simulink model "spacecraft_model_old"  (R2017a)
settings: Solver=VariableStepAuto  StartTime=0.0  StopTime=sim_time  RelTol=1e-3
StopFcn:
  | start_animation
values from neighbouring files (symbols this model uses):
  Ap = 0.1*0.2    (= 0.02)    [main_old.m]    (also in setup.m)
  Cd = 2.0    (= 2)    [main_old.m]    (also in mon_main.m = 2.2; orbit.m = 2.2; setup.m)
  Cp = 1.6    [main_old.m]    (also in setup.m)
  g_chap = q_chap(1:3)'    [main_old.m]    (also in setup.m = [0 0 0]; start_simulation_old.m)
  g_chap_data = []    [main_old.m]    (also in start_simulation_old.m)
  h_0 = [0,0,0]'    [main_old.m]    (also in setup.m)
  h_chap = [0.01 0.01 0.01]    [main_old.m]    (also in main_old2.m = [.0005;.0005;.0005]; setup.m)
  I = diag([I_x,I_y,I_z])    [main_old.m]    (also in setup.m)
  i_max = 0.25    [main_old.m]    (also in setup.m)
  K_data = []    [main_old.m]    (also in start_simulation_old.m)
  m_dipoleDist = [0.0001; -0.0001; 0.0005]'    [main_old.m]    (also in setup.m)
  mx_max = 0.2    [main_old.m]    (also in setup.m)
  my_max = 0.2    [main_old.m]    (also in setup.m)
  mz_max = 0.2    [main_old.m]    (also in setup.m)
  Pp = 4.5*10^-6    (= 4.5e-06)    [main_old.m]    (also in setup.m)
  q_0 = euler2quat(euler_0)'    [main_old.m]    (also in setup.m; start_simulation_old.m = euler2quat(euler_o_b_0)')
  r = 1+k    [anim_old.m]    (also in main_old.m = [0.005,0.001,0.001]'; orbit_J2.m = norm(y(1:3)); orbit_spherical.m = norm(y(1:3)); setup.m = [0.005,0.001,0.001]')
  rho = 42.418*10^-11    (= 4.2418e-10)    [main_old.m]    (also in mon_main.m = 2.6e-12; orbit.m = 2.6e-12; setup.m)
  sample_time = step_time*lqr_step    (= 0.1)    [main_old.m]    (also in start_simulation_old.m = 1)
  v0 = 2*pi*r_o/T_o    [main_old.m]    (also in setup.m)
  vx_max = 2.5    [main_old.m]    (also in setup.m)
  vy_max = 2.5    [main_old.m]    (also in setup.m)
  vz_max = 5    [main_old.m]    (also in setup.m)
  W = wheels_config.distr_matrix    [main_old.m]    (also in setup.m)
  w_0 = sqrt(mu/(r_o^3))    [main_old.m]    (also in setup.m)
  w_b_ib_0 = w0 + w_o_ib    [main_old.m]    (also in setup.m; start_simulation_old.m = w_o_b_0 + w_o_ib)
  w_chap = [0 0 0]    [main_old.m]    (also in main_old2.m = [0;0;0]; setup.m)
  w_o_io = [0,w_0,0]'    [main_old.m]    (also in setup.m; start_simulation_old.m = [0;w_0;0])
undefined symbols (not defined in the file or in its folder): box300, boy300, boz300, C, Ki, Kr, time300
libraries: vrlib x6, simulink x1
settings Model: Creator=Araawn  LastModifiedBy=Araawn

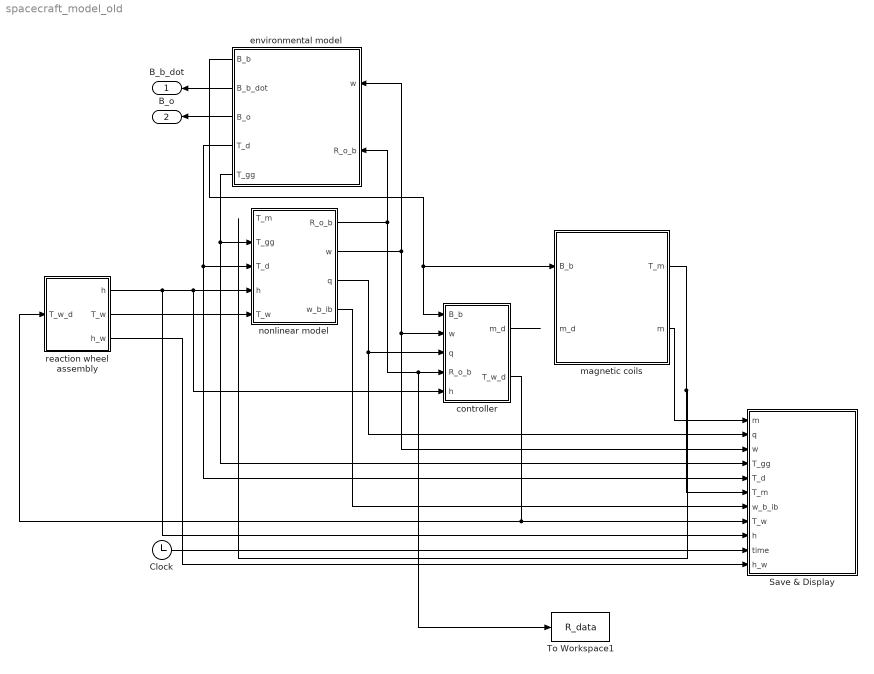
== system spacecraft_model_old ==
  Clock : Clock
  Save & Display : Subsystem
  To Workspace1 : ToWorkspace  VariableName=R_data  SaveFormat=Timeseries  SampleTime=-1
  controller : Subsystem
  environmental model : Subsystem
  magnetic coils : Subsystem
  "nonlinear model " : Subsystem
  reaction wheel assembly : Subsystem
  B_b_dot : Outport
  B_o : Outport  Port=2
  wires:
  environmental model/5(T_gg) -> "nonlinear model "/2("T_gg "), Save & Display/4(T_gg)
  environmental model/4(T_d) -> "nonlinear model "/3(T_d), Save & Display/5(T_d)
  "nonlinear model "/2(w) -> environmental model/1(w), Save & Display/3(w), controller/2(w)
  "nonlinear model "/1(R_o_b) -> To Workspace1/1, controller/4(R_o_b), environmental model/2(R_o_b)
  Clock/1 -> Save & Display/10(time)
  "nonlinear model "/3("q ") -> Save & Display/2(q), controller/3(q)
  environmental model/3(B_o) -> B_o/1
  environmental model/2(B_b_dot) -> B_b_dot/1
  "nonlinear model "/4(w_b_ib) -> Save & Display/7(w_b_ib)
  reaction wheel assembly/1(h) -> Save & Display/9(h), "nonlinear model "/4(h), controller/5(h)
  controller/2(T_w_d) -> reaction wheel assembly/1(T_w_d), Save & Display/8(T_w)
  magnetic coils/2(m) -> Save & Display/1(m)
  environmental model/1(B_b) -> magnetic coils/1(B_b), controller/1(B_b)
  controller/1(m_d) -> ?
  magnetic coils/1(T_m) -> Save & Display/6(T_m)
  reaction wheel assembly/2(T_w) -> "nonlinear model "/5(T_w)
  reaction wheel assembly/3(h_w) -> Save & Display/11(h_w)

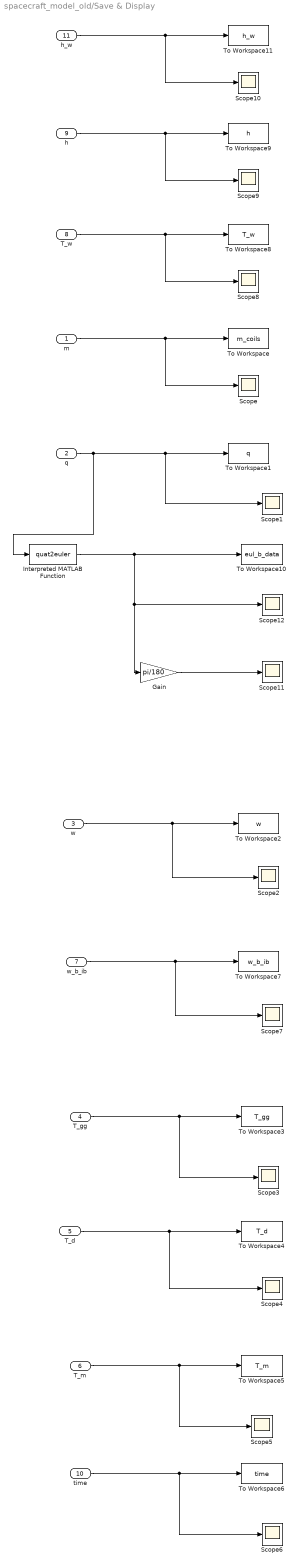
== system spacecraft_model_old/Save & Display ==
  m : Inport
  q : Inport  Port=2
  w : Inport  Port=3
  T_gg : Inport  Port=4
  T_d : Inport  Port=5
  T_m : Inport  Port=6
  w_b_ib : Inport  Port=7
  T_w : Inport  Port=8
  h : Inport  Port=9
  time : Inport  Port=10
  h_w : Inport  Port=11
  Gain : Gain  Gain=pi/180
  Interpreted MATLAB Function : MATLABFcn  MATLABFcn=quat2euler
  Scope{,1..12} (13 alike) : Scope
  To Workspace : ToWorkspace  VariableName=m_coils  SaveFormat=Timeseries  SampleTime=-1
  To Workspace1 : ToWorkspace  VariableName=q  SaveFormat=Timeseries  SampleTime=-1
  To Workspace10 : ToWorkspace  VariableName=eul_b_data  SaveFormat=Timeseries  SampleTime=-1
  To Workspace11 : ToWorkspace  VariableName=h_w  SaveFormat=Timeseries  SampleTime=-1
  To Workspace2 : ToWorkspace  VariableName=w  SaveFormat=Timeseries  SampleTime=-1
  To Workspace3 : ToWorkspace  VariableName=T_gg  SaveFormat=Timeseries  SampleTime=-1
  To Workspace4 : ToWorkspace  VariableName=T_d  SaveFormat=Timeseries  SampleTime=-1
  To Workspace5 : ToWorkspace  VariableName=T_m  SaveFormat=Timeseries  SampleTime=-1
  To Workspace6 : ToWorkspace  VariableName=time  SaveFormat=Timeseries  SampleTime=-1
  To Workspace7 : ToWorkspace  VariableName=w_b_ib  SaveFormat=Timeseries  SampleTime=-1
  To Workspace8 : ToWorkspace  VariableName=T_w  SaveFormat=Timeseries  SampleTime=-1
  To Workspace9 : ToWorkspace  VariableName=h  SaveFormat=Timeseries  SampleTime=-1
  wires:
  m/1 -> Scope/1, To Workspace/1
  q/1 -> Interpreted MATLAB Function/1, Scope1/1, To Workspace1/1
  w/1 -> Scope2/1, To Workspace2/1
  T_gg/1 -> Scope3/1, To Workspace3/1
  T_d/1 -> Scope4/1, To Workspace4/1
  T_m/1 -> Scope5/1, To Workspace5/1
  time/1 -> Scope6/1, To Workspace6/1
  w_b_ib/1 -> Scope7/1, To Workspace7/1
  T_w/1 -> Scope8/1, To Workspace8/1
  h/1 -> Scope9/1, To Workspace9/1
  Interpreted MATLAB Function/1 -> To Workspace10/1, Scope12/1, Gain/1
  Gain/1 -> Scope11/1
  h_w/1 -> Scope10/1, To Workspace11/1

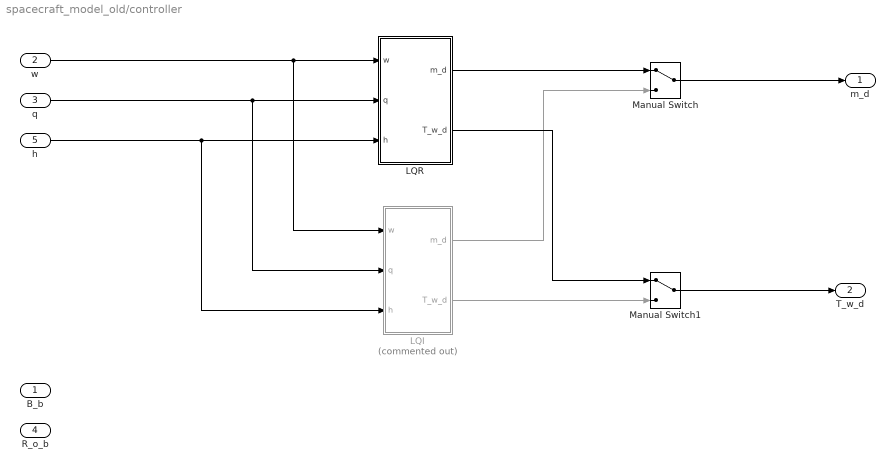
== system spacecraft_model_old/controller ==
  B_b : Inport
  w : Inport  Port=2
  q : Inport  Port=3
  R_o_b : Inport  Port=4
  h : Inport  Port=5
  LQI : Subsystem  Commented=on
  LQR : Subsystem
  Manual Switch : ManualSwitch
  Manual Switch1 : ManualSwitch
  m_d : Outport
  T_w_d : Outport  Port=2
  wires:
  w/1 -> LQR/1(w), LQI/1(w)
  q/1 -> LQR/2(q), LQI/2(q)
  h/1 -> LQR/3(h), LQI/3(h)
  LQR/1(m_d) -> Manual Switch/1
  LQI/1(m_d) -> Manual Switch/2
  Manual Switch/1 -> m_d/1
  LQI/2(T_w_d) -> Manual Switch1/2
  LQR/2(T_w_d) -> Manual Switch1/1
  Manual Switch1/1 -> T_w_d/1

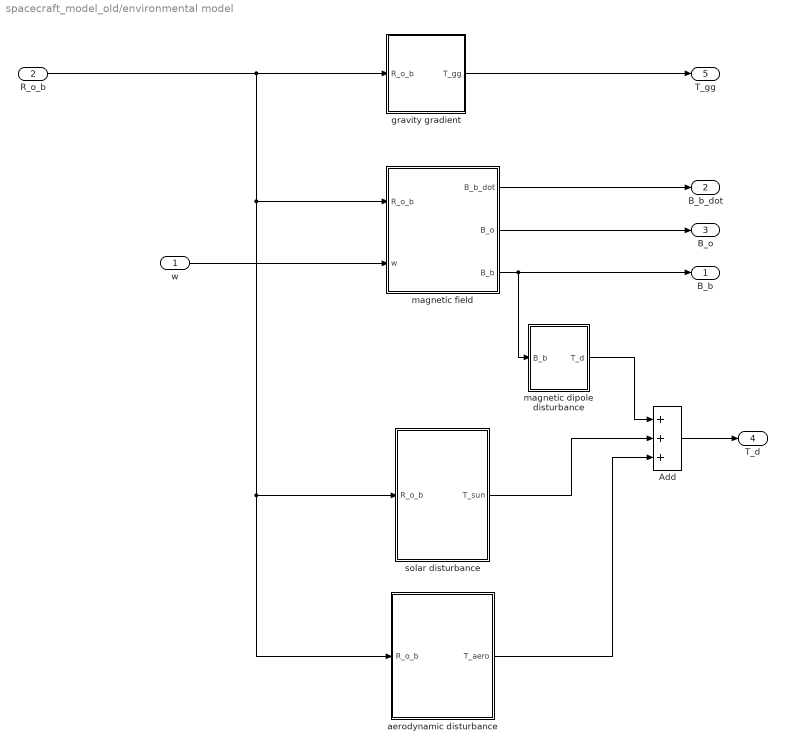
== system spacecraft_model_old/environmental model ==
  w : Inport
  R_o_b : Inport  Port=2
  Add : Sum  Inputs=+++
  aerodynamic disturbance : Subsystem
  gravity gradient : Subsystem
  magnetic dipole disturbance : Subsystem
  magnetic field : Subsystem
  solar disturbance : Subsystem
  B_b : Outport
  B_b_dot : Outport  Port=2
  B_o : Outport  Port=3
  T_d : Outport  Port=4
  T_gg : Outport  Port=5
  wires:
  magnetic field/3(B_b) -> B_b/1, magnetic dipole disturbance/1(B_b)
  Add/1 -> T_d/1
  magnetic dipole disturbance/1(T_d) -> Add/1
  magnetic field/2(B_o) -> B_o/1
  gravity gradient/1(T_gg) -> T_gg/1
  solar disturbance/1(T_sun) -> Add/2
  aerodynamic disturbance/1(T_aero) -> Add/3
  magnetic field/1(B_b_dot) -> B_b_dot/1
  R_o_b/1 -> gravity gradient/1(R_o_b), solar disturbance/1(R_o_b), aerodynamic disturbance/1(R_o_b), magnetic field/1(R_o_b)
  w/1 -> magnetic field/2(w)

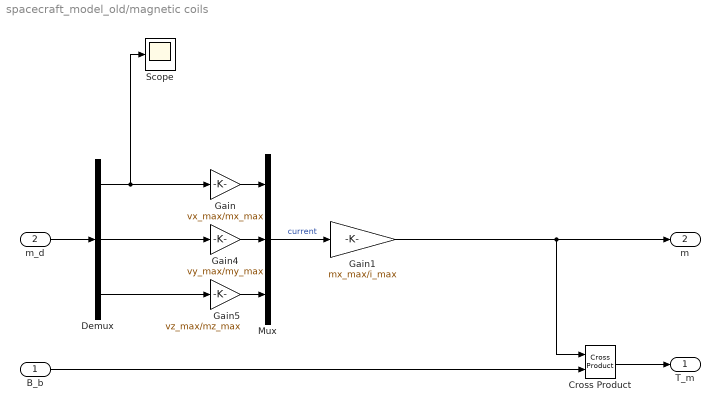
== system spacecraft_model_old/magnetic coils ==
  B_b : Inport
  m_d : Inport  Port=2
  Cross Product : vrlib/Utilities/Cross Product
      settings: SourceProductBaseCode=VR
  Demux : Demux  Outputs=3
  Gain : Gain  Gain=vx_max/mx_max
  Gain1 : Gain  Gain=mx_max/i_max
  Gain4 : Gain  Gain=vy_max/my_max
  Gain5 : Gain  Gain=vz_max/mz_max
  Mux : Mux  Inputs=3
  Scope : Scope
  T_m : Outport
  m : Outport  Port=2
  wires:
  Demux/1 -> Gain/1, Scope/1
  B_b/1 -> Cross Product/2
  Mux/1 -> Gain1/1  "current"
  Demux/3 -> Gain5/1
  Cross Product/1 -> T_m/1
  Demux/2 -> Gain4/1
  m_d/1 -> Demux/1
  Gain1/1 -> m/1, Cross Product/1
  Gain/1 -> Mux/1
  Gain5/1 -> Mux/3
  Gain4/1 -> Mux/2

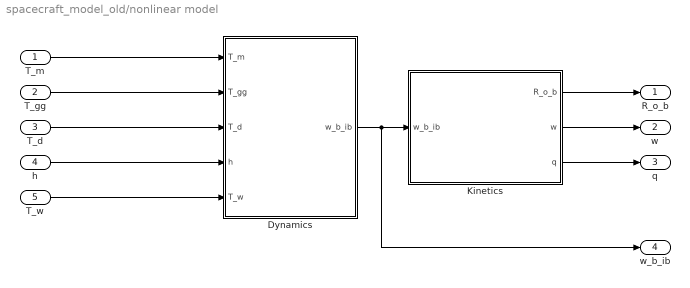
== system spacecraft_model_old/nonlinear model  ==
  T_m : Inport
  "T_gg " : Inport  Port=2
  T_d : Inport  Port=3
  h : Inport  Port=4
  T_w : Inport  Port=5
  "Dynamics " : Subsystem
  Kinetics : Subsystem
  R_o_b : Outport
  w : Outport  Port=2
  "q " : Outport  Port=3
  w_b_ib : Outport  Port=4
  wires:
  T_m/1 -> "Dynamics "/1(T_m)
  "T_gg "/1 -> "Dynamics "/2(T_gg)
  T_d/1 -> "Dynamics "/3(T_d)
  Kinetics/3(q) -> "q "/1
  Kinetics/1(R_o_b) -> R_o_b/1
  Kinetics/2(w) -> w/1
  "Dynamics "/1(w_b_ib) -> Kinetics/1("w_b_ib "), w_b_ib/1
  h/1 -> "Dynamics "/4(h)
  T_w/1 -> "Dynamics "/5(T_w)

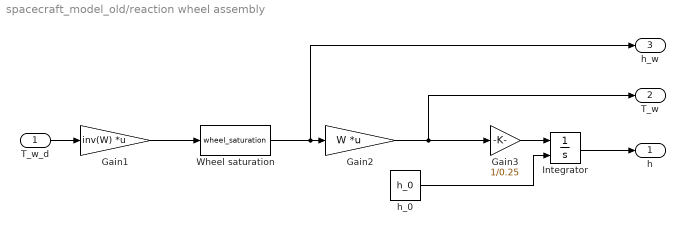
== system spacecraft_model_old/reaction wheel assembly ==
  T_w_d : Inport
  Gain1 : Gain  Gain=inv(W)  Multiplication=Matrix(K*u)
  Gain2 : Gain  Gain=W  Multiplication=Matrix(K*u)
  Gain3 : Gain  Gain=1/0.25
  Integrator : Integrator  InitialConditionSource=external
  Wheel saturation : MATLABFcn  MATLABFcn=wheel_saturation  Output1D=off
  h_0 : Constant  Value=h_0  VectorParams1D=off
  h : Outport
  T_w : Outport  Port=2
  h_w : Outport  Port=3
  wires:
  T_w_d/1 -> Gain1/1
  Gain3/1 -> Integrator/1
  h_0/1 -> Integrator/2
  Integrator/1 -> h/1
  Wheel saturation/1 -> h_w/1, Gain2/1
  Gain2/1 -> Gain3/1, T_w/1
  Gain1/1 -> Wheel saturation/1

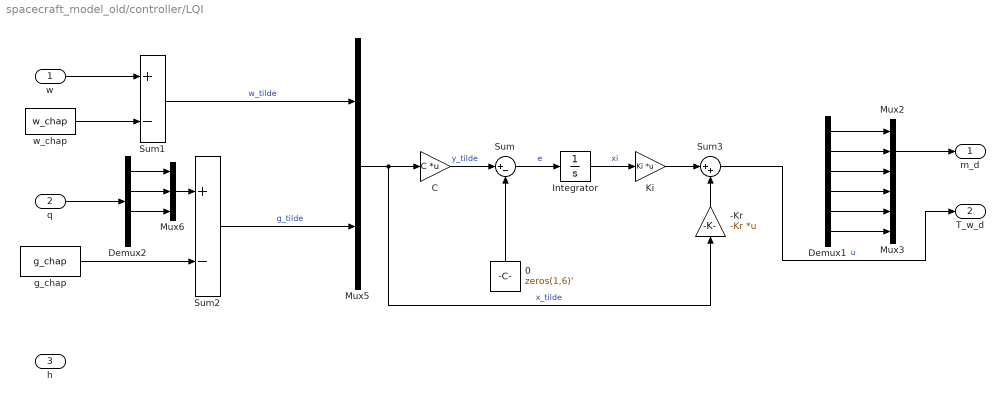
== system spacecraft_model_old/controller/LQI ==
  w : Inport
  q : Inport  Port=2
  h : Inport  Port=3
  -Kr : Gain  Gain=-Kr  Multiplication=Matrix(K*u)
  0 : Constant  Value=zeros(1,6)'
  C : Gain  Gain=C  Multiplication=Matrix(K*u)
  Demux1 : Demux  Outputs=6
  Demux2 : Demux
  Integrator : Integrator
  Ki : Gain  Gain=Ki  Multiplication=Matrix(K*u)
  Mux2 : Mux  Inputs=3
  Mux3 : Mux  Inputs=3
  Mux5 : Mux  Inputs=2
  Mux6 : Mux  Inputs=3
  Sum : Sum  Inputs=|+-
  Sum1 : Sum  Inputs=+-
  Sum2 : Sum  Inputs=+-
  Sum3 : Sum  Inputs=|++
  g_chap : Constant  Value=g_chap
  w_chap : Constant  Value=w_chap
  m_d : Outport
  T_w_d : Outport  Port=2
  wires:
  w/1 -> Sum1/1
  q/1 -> Demux2/1
  Demux1/1 -> Mux2/1
  Demux1/2 -> Mux2/2
  Demux1/3 -> Mux2/3
  Demux1/5 -> Mux3/2
  Demux1/6 -> Mux3/3
  Demux1/4 -> Mux3/1
  g_chap/1 -> Sum2/2
  w_chap/1 -> Sum1/2
  Integrator/1 -> Ki/1  "xi"
  Sum3/1 -> T_w_d/1  "u"
  Sum/1 -> Integrator/1  "e"
  Mux6/1 -> Sum2/1
  Demux2/1 -> Mux6/1
  Demux2/2 -> Mux6/2
  Demux2/3 -> Mux6/3
  Sum1/1 -> Mux5/1  "w_tilde"
  Sum2/1 -> Mux5/2  "g_tilde"
  Mux2/1 -> m_d/1
  Mux5/1 -> -Kr/1, C/1  "x_tilde"
  0/1 -> Sum/2
  C/1 -> Sum/1  "y_tilde"
  Ki/1 -> Sum3/1
  -Kr/1 -> Sum3/2

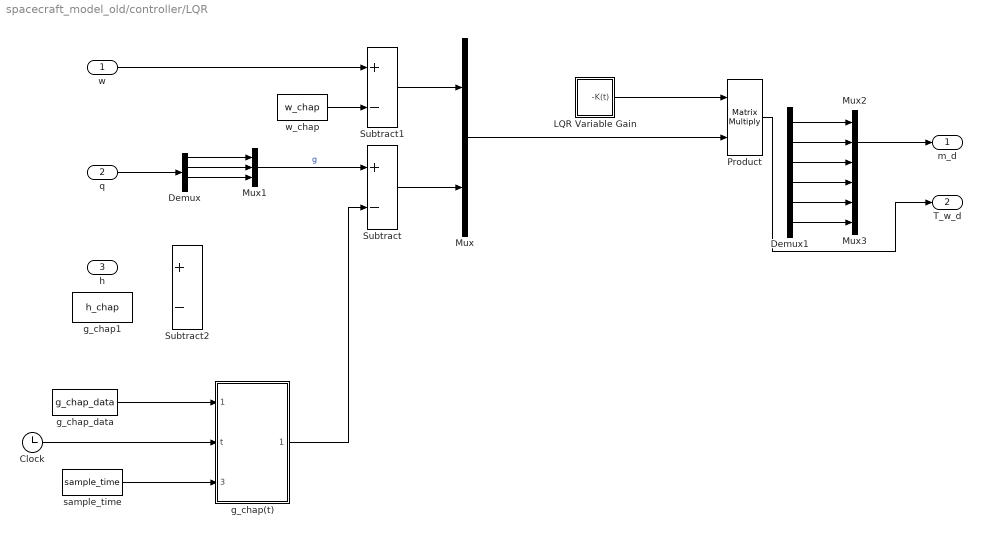
== system spacecraft_model_old/controller/LQR ==
  w : Inport
  q : Inport  Port=2
  h : Inport  Port=3
  Clock : Clock
  Demux : Demux
  Demux1 : Demux  Outputs=6
  LQR Variable Gain : Subsystem
  Mux : Mux  Inputs=2
  Mux1 : Mux  Inputs=3
  Mux2 : Mux  Inputs=3
  Mux3 : Mux  Inputs=3
  Product : Product  Multiplication=Matrix(*)
  Subtract : Sum  Inputs=+-
  Subtract1 : Sum  Inputs=+-
  Subtract2 : Sum  Inputs=+-
  g_chap(t) : MATLAB Function  TreatAsAtomicUnit=on
  g_chap1 : Constant  Value=h_chap
  g_chap_data : Constant  Value=g_chap_data
  sample_time : Constant  Value=sample_time
  w_chap : Constant  Value=w_chap
  m_d : Outport
  T_w_d : Outport  Port=2
  wires:
  Product/1 -> T_w_d/1
  Subtract/1 -> Mux/2
  q/1 -> Demux/1
  Demux1/3 -> Mux2/3
  Demux1/4 -> Mux3/1
  w/1 -> Subtract1/1
  Demux/2 -> Mux1/2
  Demux/3 -> Mux1/3
  Demux1/2 -> Mux2/2
  Mux/1 -> Product/2
  Demux/1 -> Mux1/1
  Demux1/6 -> Mux3/3
  Demux1/5 -> Mux3/2
  w_chap/1 -> Subtract1/2
  Demux1/1 -> Mux2/1
  Mux1/1 -> Subtract/1  "g"
  Mux2/1 -> m_d/1
  g_chap(t)/1(g_chap) -> Subtract/2
  Subtract1/1 -> Mux/1
  LQR Variable Gain/1(-K(t)) -> Product/1
  Clock/1 -> g_chap(t)/2(t)
  g_chap_data/1 -> g_chap(t)/1(g_chap_data)
  sample_time/1 -> g_chap(t)/3(sample_time)

== system spacecraft_model_old/environmental model/aerodynamic disturbance ==
  R_o_b : Inport
  Constant : Constant  Value=r
  Constant1 : Constant  Value=[-1;0;0]
  Cross Product : vrlib/Utilities/Cross Product
      settings: SourceProductBaseCode=VR
  Gain : Gain  Gain=0.5*rho*v0^2*Cd*Ap  Multiplication=Matrix(K*u)
  Product : Product  Multiplication=Matrix(*)
  T_aero : Outport
  wires:
  R_o_b/1 -> Product/1
  Constant1/1 -> Product/2
  Gain/1 -> Cross Product/2
  Product/1 -> Gain/1
  Cross Product/1 -> T_aero/1
  Constant/1 -> Cross Product/1

== system spacecraft_model_old/environmental model/gravity gradient ==
  R_o_b : Inport
  Constant : Constant  Value=[0,0,1]'
  Cross Product : vrlib/Utilities/Cross Product
      settings: SourceProductBaseCode=VR
  Gain : Gain  Gain=I  Multiplication=Matrix(K*u)
  Gain1 : Gain  Gain=3*w_0^2
  Product : Product  Multiplication=Matrix(*)
  T_gg : Outport
  wires:
  Constant/1 -> Product/2
  R_o_b/1 -> Product/1
  Gain1/1 -> T_gg/1
  Gain/1 -> Cross Product/2
  Cross Product/1 -> Gain1/1
  Product/1 -> Cross Product/1, Gain/1

== system spacecraft_model_old/environmental model/magnetic dipole disturbance ==
  B_b : Inport
  Constant : Constant  Value=m_dipoleDist
  Cross Product : vrlib/Utilities/Cross Product
      settings: SourceProductBaseCode=VR
  T_d : Outport
  wires:
  B_b/1 -> Cross Product/2
  Constant/1 -> Cross Product/1
  Cross Product/1 -> T_d/1

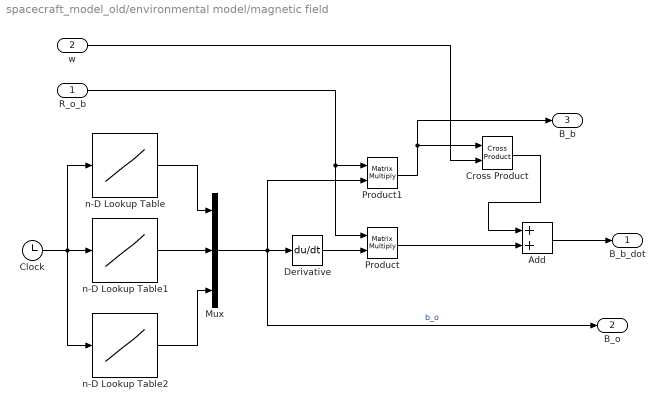
== system spacecraft_model_old/environmental model/magnetic field ==
  R_o_b : Inport
  w : Inport  Port=2
  Add : Sum
  Clock : Clock
  Cross Product : vrlib/Utilities/Cross Product
      settings: SourceProductBaseCode=VR
  Derivative : Derivative
  Mux : Mux  Inputs=3
  Product : Product  Multiplication=Matrix(*)
  Product1 : Product  Multiplication=Matrix(*)
  n-D Lookup Table : Lookup_n-D  NumberOfTableDimensions=1  LookupTableObject=B_O_x  BreakpointsForDimension1=time300  BreakpointsForDimension3=[5, 7]  Table=box300  InternalRulePriority=Speed  RndMeth=Simplest  InputSameDT=on
  n-D Lookup Table1 : Lookup_n-D  NumberOfTableDimensions=1  BreakpointsForDimension1=time300  BreakpointsForDimension3=[5, 7]  Table=boy300  InternalRulePriority=Speed  RndMeth=Simplest  InputSameDT=on
  n-D Lookup Table2 : Lookup_n-D  NumberOfTableDimensions=1  BreakpointsForDimension1=time300  BreakpointsForDimension3=[5, 7]  Table=boz300  InternalRulePriority=Speed  RndMeth=Simplest  InputSameDT=on
  B_b_dot : Outport
  B_o : Outport  Port=2
  B_b : Outport  Port=3
  wires:
  n-D Lookup Table/1 -> Mux/1
  Clock/1 -> n-D Lookup Table2/1, n-D Lookup Table1/1, n-D Lookup Table/1
  n-D Lookup Table1/1 -> Mux/2
  R_o_b/1 -> Product1/1, Product/1
  n-D Lookup Table2/1 -> Mux/3
  Add/1 -> B_b_dot/1
  Derivative/1 -> Product/2
  w/1 -> Cross Product/2
  Product1/1 -> B_b/1, Cross Product/1
  Cross Product/1 -> Add/1
  Product/1 -> Add/2
  Mux/1 -> B_o/1, Product1/2, Derivative/1  "b_o"

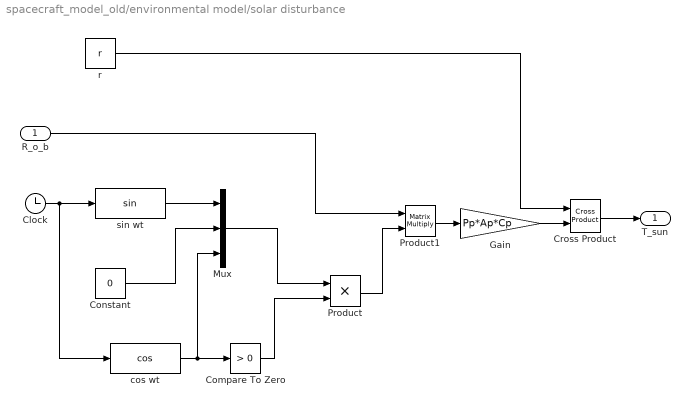
== system spacecraft_model_old/environmental model/solar disturbance ==
  R_o_b : Inport
  Clock : Clock
  Compare To Zero : simulink/Logic and Bit Operations/Compare To Zero  relop=>  OutDataTypeStr=boolean
  Constant : Constant  Value=0
  Cross Product : vrlib/Utilities/Cross Product
      settings: SourceProductBaseCode=VR
  Gain : Gain  Gain=Pp*Ap*Cp
  Mux : Mux  Inputs=3
  Product : Product
  Product1 : Product  Multiplication=Matrix(*)
  cos wt : MATLABFcn  MATLABFcn=cos
  r : Constant  Value=r
  sin wt : MATLABFcn
  T_sun : Outport
  wires:
  R_o_b/1 -> Product1/1
  Cross Product/1 -> T_sun/1
  r/1 -> Cross Product/1
  Constant/1 -> Mux/2
  Product1/1 -> Gain/1
  cos wt/1 -> Mux/3, Compare To Zero/1
  Clock/1 -> cos wt/1, sin wt/1
  sin wt/1 -> Mux/1
  Product/1 -> Product1/2
  Mux/1 -> Product/1
  Gain/1 -> Cross Product/2
  Compare To Zero/1 -> Product/2

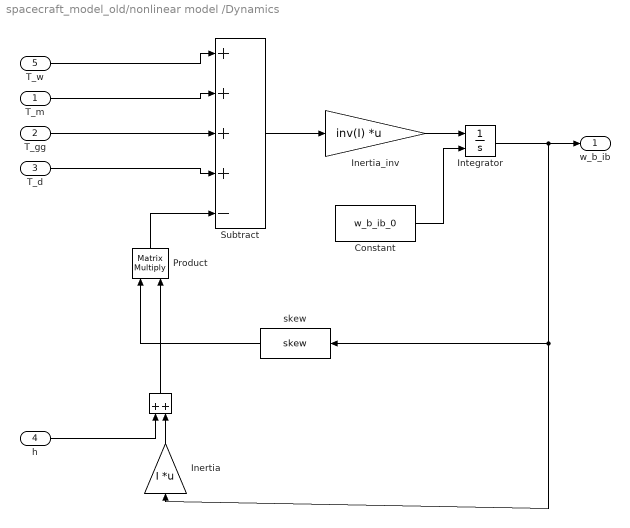
== system spacecraft_model_old/nonlinear model /Dynamics  ==
  T_m : Inport
  T_gg : Inport  Port=2
  T_d : Inport  Port=3
  h : Inport  Port=4
  T_w : Inport  Port=5
  " " : Sum
  Constant : Constant  Value=w_b_ib_0  VectorParams1D=off
  "Inertia " : Gain  Gain=I  Multiplication=Matrix(K*u)
  Inertia_inv : Gain  Gain=inv(I)  Multiplication=Matrix(K*u)
  Integrator : Integrator  InitialConditionSource=external
  Product : Product  Multiplication=Matrix(*)
  Subtract : Sum  Inputs=++++-
  skew : MATLABFcn  MATLABFcn=skew  Output1D=off
  w_b_ib : Outport
  wires:
  Constant/1 -> Integrator/2
  Subtract/1 -> Inertia_inv/1
  Integrator/1 -> "Inertia "/1, skew/1, w_b_ib/1
  T_gg/1 -> Subtract/3
  T_m/1 -> Subtract/2
  T_d/1 -> Subtract/4
  Inertia_inv/1 -> Integrator/1
  Product/1 -> Subtract/5
  " "/1 -> Product/2
  "Inertia "/1 -> " "/2
  h/1 -> " "/1
  skew/1 -> Product/1
  T_w/1 -> Subtract/1

== system spacecraft_model_old/nonlinear model /Kinetics ==
  "w_b_ib " : Inport
  Constant : Constant  Value=q_0'  VectorParams1D=off
  Integrator : Integrator  InitialConditionSource=external
  MATLAB Function : MATLAB Function  TreatAsAtomicUnit=on
  Product : Product  Multiplication=Matrix(*)
  "orbit_to_body " : Subsystem
  R_o_b : Outport
  w : Outport  Port=2
  q : Outport  Port=3
  wires:
  MATLAB Function/1(W) -> Product/1
  Constant/1 -> Integrator/2
  Product/1 -> Integrator/1
  "w_b_ib "/1 -> "orbit_to_body "/2(w_b_ib)
  "orbit_to_body "/1(w) -> w/1, Product/2
  Integrator/1 -> q/1, "orbit_to_body "/1(q), MATLAB Function/1(q)
  "orbit_to_body "/2(R_o_b) -> R_o_b/1

== system spacecraft_model_old/controller/LQR/LQR Variable Gain ==
  Clock : Clock
  Gain : Gain  Gain=-1
  K(t) : MATLAB Function  TreatAsAtomicUnit=on
  K_data : Constant  Value=K_data
  sample_time : Constant  Value=sample_time
  -K(t) : Outport
  wires:
  K_data/1 -> K(t)/1(K_data)
  K(t)/1(K) -> Gain/1
  sample_time/1 -> K(t)/3(sample_time)
  Gain/1 -> -K(t)/1
  Clock/1 -> K(t)/2(t)

== system spacecraft_model_old/nonlinear model /Kinetics/orbit_to_body  ==
  q : Inport
  w_b_ib : Inport  Port=2
  Constant : Constant  Value=w_o_io  VectorParams1D=off
  Product : Product  Multiplication=Matrix(*)
  Rquat : MATLABFcn  MATLABFcn=Rquat  Output1D=off
  Sum : Sum  Inputs=|+-
  w : Outport
  R_o_b : Outport  Port=2
  wires:
  Sum/1 -> w/1
  Constant/1 -> Product/2
  q/1 -> Rquat/1
  Product/1 -> Sum/2
  w_b_ib/1 -> Sum/1
  Rquat/1 -> R_o_b/1, Product/1

== matlab function spacecraft_model_old/nonlinear model /Kinetics/MATLAB Function ==
  data: q input; W output
function W = Wq(q)
W = 0.5*[q(4) -q(3) q(2);
q(3) q(4) -q(1);
-q(2) q(1) q(4);
-q(1) -q(2) -q(3)];
end

== matlab function spacecraft_model_old/controller/LQR/LQR Variable Gain/K(t) ==
  data: K_data input; K output; t input; sample_time input
function K = K_t(K_data,t,sample_time)
    step=floor(t/sample_time)+1;
    K=K_data(1:3,6*step-5:6*step);
end

== matlab function spacecraft_model_old/controller/LQR/g_chap(t) ==
  data: g_chap_data input; g_chap output; t input; sample_time input
function g_chap = g_chap_t(g_chap_data,t,sample_time)
    step=floor(t/sample_time)+1;
    g_chap=g_chap_data(:,step);
end
